simulink model "Wahadlo_clean"  (R2015a)
settings: Solver=ode5  SolverMode=SingleTasking  StartTime=0.0  StopTime=9999  FixedStep=0.01  RelTol=1e-3  AbsTol=1e-6
undefined symbols (not defined in the file): RTDAC4PCIBaseAddress
settings Model: SimulationMode=external  ExtModeTrigDuration=12000  ExtModeTrigLevel=0.400000  Creator=jims  LastModifiedBy=Lab
settings DataIOCC: ExternalInput=[]  InitialState=[]  LimitDataPoints=off  MaxDataPoints=5000  SignalLoggingSaveFormat=ModelDataLogs  SaveOutput=off  SaveTime=off  SignalLoggingName=sigsOut
settings OptimizationCC: BooleanDataType=off  ExpressionDepthLimit=2147483647  InitFltsAndDblsToZero=on
settings DebuggingCC: SaveWithParameterizedLinksMsg=none  UnderspecifiedInitializationDetection=Classic  MergeDetectMultiDrivingBlocksExec=none  SignalResolutionControl=TryResolveAllWithWarning  MultiTaskDSMMsg=warning  MultiTaskCondExecSysMsg=none  IntegerOverflowMsg=none  FcnCallInpInsideContextMsg=UseLocalSettings  StateNameClashWarn=warning  IntegerSaturationMsg=none
settings HardwareCC: ProdBitPerLong=64  ProdBitPerPointer=64  ProdIntDivRoundTo=Zero  ProdEndianess=LittleEndian  ProdWordSize=64  ProdHWDeviceType=Intel->x86-64  TargetBitPerLong=64  TargetBitPerPointer=64  TargetIntDivRoundTo=Zero  TargetEndianess=LittleEndian  TargetWordSize=64  TargetHWDeviceType=Intel->x86-64
settings RTWCC: SystemTargetFile=rtwin.tlc  TemplateMakefile=RTDAC_win.tmf  Description=Real-Time Windows Target
settings RTWinTargetCC: TargetFcnLib=ansi_tfl_tmw.mat  TargetPreCompLibLocation=C:\Program Files\MATLAB\R2015aSP1\toolbox\sldrt\lib\win64  ModelReferenceCompliant=off  CompOptLevelCompliant=off

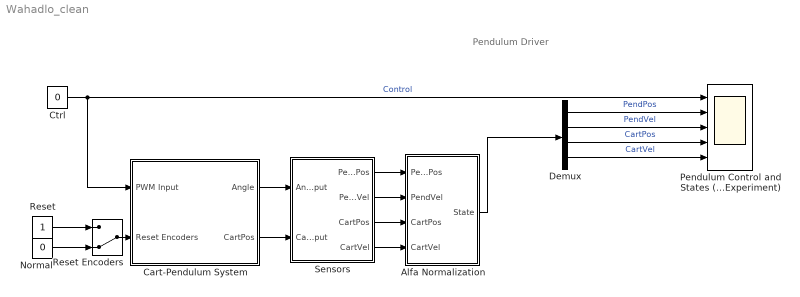
== system Wahadlo_clean ==
  note: Pendulum
      | Driver
  Alfa Normalization : Subsystem  mask(Choose mode:){pos=Inverted Pendulum}
      mask prompts: pos "Choose mode:"
      mask TypeOptions pos: Inverted Pendulum | Crane Controller
  Cart-Pendulum System : Subsystem  mask{BaseAddress=RTDAC4PCIBaseAddress(-1,-1), T0=0.01}
      mask prompts: BaseAddress "Base Address:"; T0 "Sampling Period:"
      mask Display: plot( [0.725 0.725], [1.05 0.375], 0.725+0.05*sin([0:0.5:7]), 0.325+0.05*cos([0:0.5:7]), [-0.3 -0.3], [-0.3 -0.3], [1.8 1.8], [1.8 1.8], [0.1 1.4], [0.95 0.95], [0.1 1.4], [0.92 0.92], [0.65 0.8], [1 1], [0.65 0.8], [1.1 1.1], [0.65 0.65], [1.1 1], [0.8 0.8], [1 1.1] )
  Ctrl : Constant  Value=0
  Demux : Demux
  Normal : Constant  Value=0
  Pendulum Control and States (Experiment) : Scope  NumInputPorts=5
      settings: TimeRange=10  YMin=-1~-4~-0.2~-0.9765~-1  YMax=1~4~0.2~-0.8835~1  SaveName=P1_Data  MaxDataPoints=50000
  Reset : Constant
  Reset Encoders : ManualSwitch  CurrentSetting=0
  Sensors : Subsystem  mask(PENDULUM Output){T0=0.01}
      mask prompts: T0 "Sample Time"
      mask help: PCL-812 PG Device Driver
  wires:
  Reset Encoders/1 -> Cart-Pendulum System/2(Reset Encoders)
  Normal/1 -> Reset Encoders/2
  Reset/1 -> Reset Encoders/1
  Sensors/1(PendPos) -> Alfa Normalization/1(PendPos)
  Sensors/2(PendVel) -> Alfa Normalization/2(PendVel)
  Sensors/3(CartPos) -> Alfa Normalization/3(CartPos)
  Sensors/4(CartVel) -> Alfa Normalization/4(CartVel)
  Cart-Pendulum System/1(Angle) -> Sensors/1(AngleInput)
  Cart-Pendulum System/2(CartPos) -> Sensors/2(CartPosInput)
  Ctrl/1 -> Cart-Pendulum System/1(PWM Input), Pendulum Control and States (Experiment)/1  "Control"
  Alfa Normalization/1(State) -> Demux/1
  Demux/4 -> Pendulum Control and States (Experiment)/5  "CartVel"
  Demux/3 -> Pendulum Control and States (Experiment)/4  "CartPos"
  Demux/2 -> Pendulum Control and States (Experiment)/3  "PendVel"
  Demux/1 -> Pendulum Control and States (Experiment)/2  "PendPos"

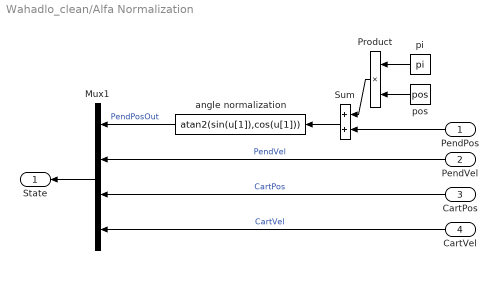
== system Wahadlo_clean/Alfa Normalization ==
  PendPos : Inport
  PendVel : Inport  Port=2
  CartPos : Inport  Port=3
  CartVel : Inport  Port=4
  Mux1 : Mux
  Product : Product  SaturateOnIntegerOverflow=on  InputSameDT=on  OutDataTypeStr=Inherit: Same as first input
  Sum : Sum  SaturateOnIntegerOverflow=on  InputSameDT=on  OutDataTypeStr=Inherit: Same as first input
  angle normalization : Fcn  Expr=atan2(sin(u[1]),cos(u[1]))
  pi : Constant  Value=pi
  pos : Constant  Value=pos
  State : Outport  InitialOutput=0
  wires:
  angle normalization/1 -> Mux1/1  "PendPosOut"
  PendVel/1 -> Mux1/2  "PendVel"
  CartVel/1 -> Mux1/4  "CartVel"
  CartPos/1 -> Mux1/3  "CartPos"
  Mux1/1 -> State/1
  Sum/1 -> angle normalization/1
  PendPos/1 -> Sum/2
  pi/1 -> Product/1
  pos/1 -> Product/2
  Product/1 -> Sum/1

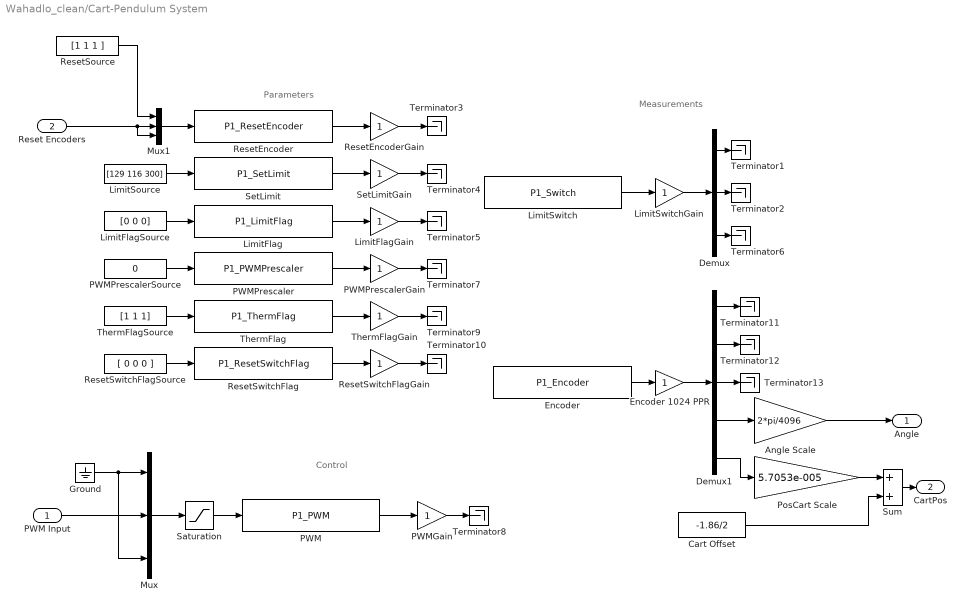
== system Wahadlo_clean/Cart-Pendulum System ==
  note: Measurements
  note: Control
  note: Parameters
  PWM Input : Inport
  Reset Encoders : Inport  Port=2
  Angle Scale : Gain  Gain=2*pi/4096  OutDataTypeStr=Inherit: Same as input  ParamDataTypeStr=Inherit: Same as input
  Cart Offset : Constant  Value=-1.86/2
  Demux : Demux  Outputs=3
  Demux1 : Demux  Outputs=5
  Encoder : S-Function  FunctionName=P1_Encoder  Parameters=BaseAddress, T0
  Encoder 1024 PPR : Gain  SaturateOnIntegerOverflow=on  OutDataTypeStr=Inherit: Same as input  ParamDataTypeStr=Inherit: Same as input
  Ground : Ground
  LimitFlag : S-Function  FunctionName=P1_LimitFlag  Parameters=BaseAddress, T0
  LimitFlagGain : Gain  SaturateOnIntegerOverflow=on  OutDataTypeStr=Inherit: Same as input  ParamDataTypeStr=Inherit: Same as input
  LimitFlagSource : Constant  Value=[0 0 0]
  LimitSource : Constant  Value=[129 116 300]
  LimitSwitch : S-Function  FunctionName=P1_Switch  Parameters=BaseAddress, T0
  LimitSwitchGain : Gain  SaturateOnIntegerOverflow=on  OutDataTypeStr=Inherit: Same as input  ParamDataTypeStr=Inherit: Same as input
  Mux : Mux  Inputs=3
  Mux1 : Mux  Inputs=[3 1 1]
  PWM : S-Function  FunctionName=P1_PWM  Parameters=BaseAddress, T0
  PWMGain : Gain  SaturateOnIntegerOverflow=on  OutDataTypeStr=Inherit: Same as input  ParamDataTypeStr=Inherit: Same as input
  PWMPrescaler : S-Function  FunctionName=P1_PWMPrescaler  Parameters=BaseAddress, T0
  PWMPrescalerGain : Gain  SaturateOnIntegerOverflow=on  OutDataTypeStr=Inherit: Same as input  ParamDataTypeStr=Inherit: Same as input
  PWMPrescalerSource : Constant  Value=0
  PosCart Scale : Gain  Gain=5.7053e-005  OutDataTypeStr=Inherit: Same as input  ParamDataTypeStr=Inherit: Same as input
  ResetEncoder : S-Function  FunctionName=P1_ResetEncoder  Parameters=BaseAddress, T0
  ResetEncoderGain : Gain  SaturateOnIntegerOverflow=on  OutDataTypeStr=Inherit: Same as input  ParamDataTypeStr=Inherit: Same as input
  ResetSource : Constant  Value=[1 1 1 ]
  "ResetSwitchFlag " : S-Function  FunctionName=P1_ResetSwitchFlag  Parameters=BaseAddress, T0
  ResetSwitchFlagGain : Gain  SaturateOnIntegerOverflow=on  OutDataTypeStr=Inherit: Same as input  ParamDataTypeStr=Inherit: Same as input
  ResetSwitchFlagSource : Constant  Value=[ 0 0 0 ]
  Saturation : Saturate
  SetLimit : S-Function  FunctionName=P1_SetLimit  Parameters=BaseAddress, T0
  SetLimitGain : Gain  SaturateOnIntegerOverflow=on  OutDataTypeStr=Inherit: Same as input  ParamDataTypeStr=Inherit: Same as input
  Sum : Sum  SaturateOnIntegerOverflow=on  InputSameDT=on  OutDataTypeStr=Inherit: Same as first input
  Terminator{1..13} (13 alike) : Terminator
  "ThermFlag " : S-Function  FunctionName=P1_ThermFlag  Parameters=BaseAddress, T0
  ThermFlagGain : Gain  SaturateOnIntegerOverflow=on  OutDataTypeStr=Inherit: Same as input  ParamDataTypeStr=Inherit: Same as input
  ThermFlagSource : Constant  Value=[1 1 1]
  Angle : Outport
  CartPos : Outport  Port=2
  wires:
  Demux1/1 -> Terminator11/1
  Demux1/2 -> Terminator12/1
  Demux1/3 -> Terminator13/1
  Demux1/4 -> Angle Scale/1
  Demux1/5 -> PosCart Scale/1
  Angle Scale/1 -> Angle/1
  Demux/3 -> Terminator6/1
  Demux/2 -> Terminator2/1
  Demux/1 -> Terminator1/1
  LimitSwitchGain/1 -> Demux/1
  LimitSwitch/1 -> LimitSwitchGain/1
  Ground/1 -> Mux/1, Mux/3
  PWM Input/1 -> Mux/2
  ResetSwitchFlagGain/1 -> Terminator10/1
  ThermFlagGain/1 -> Terminator9/1
  PWMPrescalerGain/1 -> Terminator7/1
  LimitFlagGain/1 -> Terminator5/1
  SetLimitGain/1 -> Terminator4/1
  ResetEncoderGain/1 -> Terminator3/1
  ResetSwitchFlagSource/1 -> "ResetSwitchFlag "/1
  ThermFlagSource/1 -> "ThermFlag "/1
  PWMPrescalerSource/1 -> PWMPrescaler/1
  LimitFlagSource/1 -> LimitFlag/1
  LimitSource/1 -> SetLimit/1
  "ResetSwitchFlag "/1 -> ResetSwitchFlagGain/1
  "ThermFlag "/1 -> ThermFlagGain/1
  PWMPrescaler/1 -> PWMPrescalerGain/1
  LimitFlag/1 -> LimitFlagGain/1
  SetLimit/1 -> SetLimitGain/1
  ResetEncoder/1 -> ResetEncoderGain/1
  PWMGain/1 -> Terminator8/1
  PWM/1 -> PWMGain/1
  Mux/1 -> Saturation/1
  Saturation/1 -> PWM/1
  Encoder/1 -> Encoder 1024 PPR/1
  Encoder 1024 PPR/1 -> Demux1/1
  Mux1/1 -> ResetEncoder/1
  ResetSource/1 -> Mux1/1
  Reset Encoders/1 -> Mux1/2, Mux1/3
  PosCart Scale/1 -> Sum/1
  Sum/1 -> CartPos/1
  Cart Offset/1 -> Sum/2

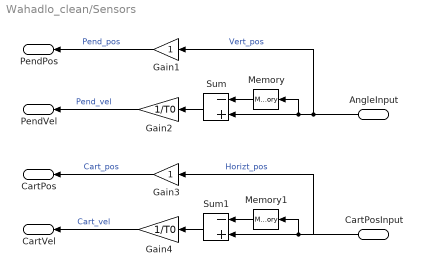
== system Wahadlo_clean/Sensors ==
  AngleInput : Inport
  CartPosInput : Inport  Port=2
  Gain1 : Gain  SaturateOnIntegerOverflow=on  OutDataTypeStr=Inherit: Same as input  ParamDataTypeStr=Inherit: Same as input
  Gain2 : Gain  Gain=1/T0  SaturateOnIntegerOverflow=on  OutDataTypeStr=Inherit: Same as input  ParamDataTypeStr=Inherit: Same as input
  Gain3 : Gain  SaturateOnIntegerOverflow=on  OutDataTypeStr=Inherit: Same as input  ParamDataTypeStr=Inherit: Same as input
  Gain4 : Gain  Gain=1/T0  SaturateOnIntegerOverflow=on  OutDataTypeStr=Inherit: Same as input  ParamDataTypeStr=Inherit: Same as input
  Memory : Memory
  Memory1 : Memory
  Sum : Sum  Inputs=-+  SaturateOnIntegerOverflow=on  InputSameDT=on  OutDataTypeStr=Inherit: Same as first input
  Sum1 : Sum  Inputs=-+  SaturateOnIntegerOverflow=on  InputSameDT=on  OutDataTypeStr=Inherit: Same as first input
  PendPos : Outport  InitialOutput=0
  PendVel : Outport  Port=2  InitialOutput=0
  CartPos : Outport  Port=3  InitialOutput=0
  CartVel : Outport  Port=4  InitialOutput=0
  wires:
  Gain4/1 -> CartVel/1  "Cart_vel"
  Sum1/1 -> Gain4/1
  Memory1/1 -> Sum1/1
  Sum/1 -> Gain2/1
  Memory/1 -> Sum/1
  CartPosInput/1 -> Memory1/1, Sum1/2, Gain3/1  "Horizt_pos"
  AngleInput/1 -> Memory/1, Sum/2, Gain1/1  "Vert_pos"
  Gain2/1 -> PendVel/1  "Pend_vel"
  Gain1/1 -> PendPos/1  "Pend_pos"
  Gain3/1 -> CartPos/1  "Cart_pos"
